simulink model "interlock_deadtime"  (R2020b)
settings: Solver=FixedStepDiscrete  StartTime=0.0  StopTime=0.01  RelTol=1e-3
libraries: eePwmGeneratorTwoLevel x1, powerlib_meascontrol x1, simulink x1, hdlsllib x1
settings Model: DataTypeOverride=Off  Creator=ts  LastModifiedBy=ts
settings DataIOCC: LimitDataPoints=on  SaveOutput=off  SaveTime=off
settings OptimizationCC: BlockReduction=off  ConditionallyExecuteInputs=off  DefaultParameterBehavior=Inlined  LifeSpan=inf
settings DebuggingCC: AlgebraicLoopMsg=error  SingleTaskRateTransMsg=error  AllowSymbolicDim=off  StrictBusMsg=ErrorOnBusTreatedAsVector  SFUnexpectedBacktrackingDiag=warning  SFNoUnconditionalDefaultTransitionDiag=warning  SFExecutionAtInitializationDiag=none  ArithmeticOperatorsInVariantConditions=warning
settings HardwareCC: ProdBitPerPointer=32  ProdBitPerSizeT=32  ProdBitPerPtrDiffT=32  ProdLargestAtomicFloat=None  ProdIntDivRoundTo=Undefined  ProdEndianess=Unspecified  ProdWordSize=32  ProdHWDeviceType=ASIC/FPGA->ASIC/FPGA  ProdEqTarget=off
settings SFSimCC: SimUseLocalCustomCode=off  CustomCodeUndefinedFunction=UseInterfaceOnly
settings RTWCC: RTWUseLocalCustomCode=off
settings CodeAppCC: StateflowObjectComments=on
settings GRTTargetCC: TargetLangStandard=C89/C90 (ANSI)
settings ConfigComp: CovScope=ReferencedModels  CovMetricSettings=dw  CovSaveCumulativeToWorkspaceVar=on  CovSaveSingleToWorkspaceVar=on  CovExternalEMLEnable=off  CovSFcnEnable=off

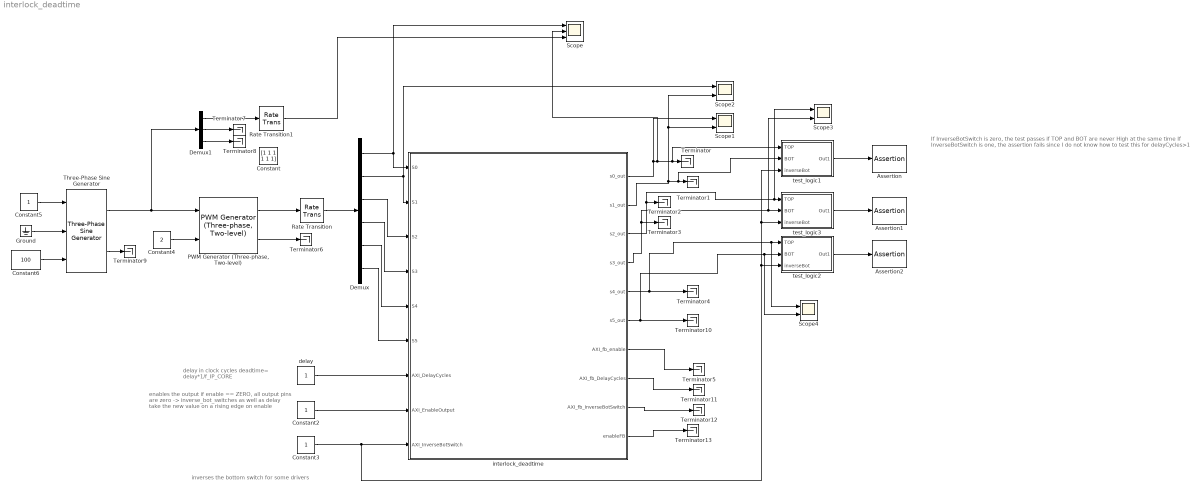
== system interlock_deadtime ==
  note: If InverseBotSwitch is zero, the test passes if TOP and BOT are never High at the same time
      | If InverseBotSwitch is one, the assertion fails since I do not know how to test this for delayCycles>1
  note: enables the output
      | if enable == ZERO, all output pins are zero
      |
      | -> inverse_bot_switches as well as delay take the
      | new value on a rising edge on enable
  note: inverses the bottom switch for some drivers
  note: delay in clock cycles
      | deadtime= delay*1/f_IP_CORE
  Assertion : Assertion
  Assertion1 : Assertion
  Assertion2 : Assertion
  Constant : Constant  Value=[1 1 1 1 1 1]  OutDataTypeStr=boolean
  Constant2 : Constant  OutDataTypeStr=boolean  SampleTime=1/100e6
  Constant3 : Constant  OutDataTypeStr=boolean  SampleTime=1/100e6
  Constant4 : Constant  Value=2  SampleTime=-1
  Constant5 : Constant  SampleTime=-1
  Constant6 : Constant  Value=100  SampleTime=-1
  Demux : Demux  Outputs=6
  Demux1 : Demux  Outputs=3
  Ground : Ground
  "PWM Generator (Three-phase, Two-level)" : eePwmGeneratorTwoLevel/PWM Generator (Three-phase, Two-level)  PWMMode=Continuous PWM (CPWM)  CPWMMode=SPWM: sinusoidal PWM  DPWMMode=60 DPWM: 60 degree discontinuous PWM  fsw=10e3  Ts=1/(100*100e3)
      settings: SourceProductBaseCode=PS
  Rate Transition : RateTransition  OutPortSampleTime=1/100e6
  Rate Transition1 : RateTransition  OutPortSampleTime=1/100e6
  Scope : Scope  NumInputPorts=3
  Scope{1..4} (4 alike) : Scope  NumInputPorts=2
  Terminator{,1..13} (14 alike) : Terminator
  Three-Phase Sine Generator : powerlib_meascontrol/Pulse & Signal Generators/Three-Phase Sine Generator  Ts=1/100e3
      settings: SourceProductBaseCode=PS
  delay : Constant  OutDataTypeStr=fixdt(0,10,0)  SampleTime=1/100e6
  interlock_deadtime : Subsystem  TreatAsAtomicUnit=on
  test_logic1 : Subsystem
  test_logic2 : Subsystem
  test_logic3 : Subsystem
  wires:
  Constant2/1 -> interlock_deadtime/8(AXI_EnableOutput)
  interlock_deadtime/1(s0_out) -> Scope/2, test_logic1/1(TOP), Terminator/1, Scope1/1
  interlock_deadtime/2(s1_out) -> Scope1/2, Scope2/2, test_logic1/2(BOT), Terminator1/1
  interlock_deadtime/3(s2_out) -> Scope3/1, test_logic3/1(TOP), Terminator2/1
  interlock_deadtime/4(s3_out) -> Scope3/2, test_logic3/2(BOT), Terminator3/1
  interlock_deadtime/5(s4_out) -> Scope4/1, test_logic2/1(TOP), Terminator4/1
  Constant4/1 -> "PWM Generator (Three-phase, Two-level)"/2
  Three-Phase Sine Generator/1 -> Demux1/1, "PWM Generator (Three-phase, Two-level)"/1
  Constant5/1 -> Three-Phase Sine Generator/1
  Constant6/1 -> Three-Phase Sine Generator/3
  Demux/1 -> Scope/1, interlock_deadtime/1(S0)
  Demux/2 -> Scope2/1, interlock_deadtime/2(S1)
  Demux/3 -> interlock_deadtime/3(S2)
  Demux/4 -> interlock_deadtime/4(S3)
  Demux/5 -> interlock_deadtime/5(S4)
  Demux/6 -> interlock_deadtime/6(S5)
  Demux1/1 -> Rate Transition1/1
  Rate Transition1/1 -> Scope/3
  Constant3/1 -> interlock_deadtime/9(AXI_InverseBotSwitch), test_logic2/3(inverseBot), test_logic3/3(inverseBot), test_logic1/3(inverseBot)
  "PWM Generator (Three-phase, Two-level)"/2 -> Terminator6/1
  Demux1/2 -> Terminator7/1
  Demux1/3 -> Terminator8/1
  Three-Phase Sine Generator/2 -> Terminator9/1
  Ground/1 -> Three-Phase Sine Generator/2
  interlock_deadtime/6(s5_out) -> Scope4/2, test_logic2/2(BOT), Terminator10/1
  interlock_deadtime/7(AXI_fb_enable) -> Terminator5/1
  interlock_deadtime/8(AXI_fb_DelayCycles) -> Terminator11/1
  interlock_deadtime/9(AXI_fb_InverseBotSwitch) -> Terminator12/1
  interlock_deadtime/10(enableFB) -> Terminator13/1
  test_logic3/1(Out1) -> Assertion1/1
  test_logic2/1(Out1) -> Assertion2/1
  test_logic1/1(Out1) -> Assertion/1
  Rate Transition/1 -> Demux/1
  "PWM Generator (Three-phase, Two-level)"/1 -> Rate Transition/1
  delay/1 -> interlock_deadtime/7(AXI_DelayCycles)

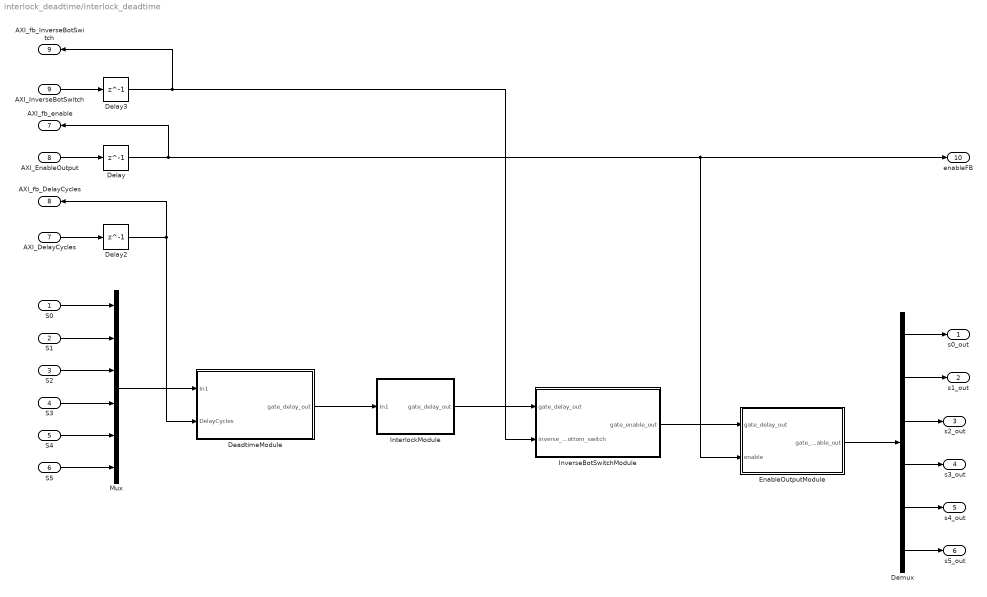
== system interlock_deadtime/interlock_deadtime ==
  S0 : Inport
  S1 : Inport  Port=2
  S2 : Inport  Port=3
  S3 : Inport  Port=4
  S4 : Inport  Port=5
  S5 : Inport  Port=6
  AXI_DelayCycles : Inport  Port=7
  AXI_EnableOutput : Inport  Port=8
  AXI_InverseBotSwitch : Inport  Port=9
  DeadtimeModule : Subsystem  TreatAsAtomicUnit=on
  Delay : Delay  DelayLength=1
  Delay2 : Delay  DelayLength=1
  Delay3 : Delay  DelayLength=1
  Demux : Demux  Outputs=6
  EnableOutputModule : Subsystem  TreatAsAtomicUnit=on
  InterlockModule : Subsystem  TreatAsAtomicUnit=on
  InverseBotSwitchModule : Subsystem  TreatAsAtomicUnit=on
  Mux : Mux  Inputs=6
  s0_out : Outport  VectorParamsAs1DForOutWhenUnconnected=off
  s1_out : Outport  Port=2  VectorParamsAs1DForOutWhenUnconnected=off
  s2_out : Outport  Port=3  VectorParamsAs1DForOutWhenUnconnected=off
  s3_out : Outport  Port=4  VectorParamsAs1DForOutWhenUnconnected=off
  s4_out : Outport  Port=5  VectorParamsAs1DForOutWhenUnconnected=off
  s5_out : Outport  Port=6  VectorParamsAs1DForOutWhenUnconnected=off
  AXI_fb_enable : Outport  Port=7  VectorParamsAs1DForOutWhenUnconnected=off
  AXI_fb_DelayCycles : Outport  Port=8  VectorParamsAs1DForOutWhenUnconnected=off
  AXI_fb_InverseBotSwitch : Outport  Port=9  VectorParamsAs1DForOutWhenUnconnected=off
  enableFB : Outport  Port=10  VectorParamsAs1DForOutWhenUnconnected=off
  wires:
  AXI_InverseBotSwitch/1 -> Delay3/1
  Delay3/1 -> InverseBotSwitchModule/2(inverse_bottom_switch), AXI_fb_InverseBotSwitch/1
  AXI_EnableOutput/1 -> Delay/1
  Delay2/1 -> AXI_fb_DelayCycles/1, DeadtimeModule/2(DelayCycles)
  Mux/1 -> DeadtimeModule/1(In1)
  DeadtimeModule/1(gate_delay_out) -> InterlockModule/1(In1)
  S0/1 -> Mux/1
  S1/1 -> Mux/2
  S2/1 -> Mux/3
  S3/1 -> Mux/4
  S4/1 -> Mux/5
  S5/1 -> Mux/6
  Demux/2 -> s1_out/1
  Demux/1 -> s0_out/1
  Demux/3 -> s2_out/1
  Demux/4 -> s3_out/1
  Demux/5 -> s4_out/1
  Demux/6 -> s5_out/1
  EnableOutputModule/1(gate_enable_out) -> Demux/1
  Delay/1 -> AXI_fb_enable/1, enableFB/1, EnableOutputModule/2(enable)
  InterlockModule/1(gate_delay_out) -> InverseBotSwitchModule/1(gate_delay_out)
  InverseBotSwitchModule/1(gate_enable_out) -> EnableOutputModule/1(gate_delay_out)
  AXI_DelayCycles/1 -> Delay2/1

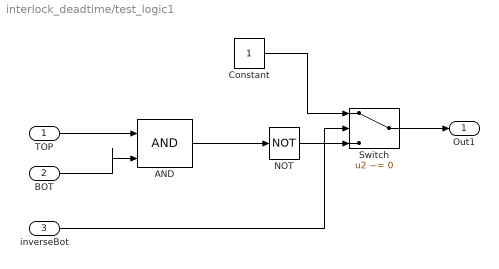
== system interlock_deadtime/test_logic1 ==
  TOP : Inport
  BOT : Inport  Port=2
  inverseBot : Inport  Port=3
  AND : Logic  IconShape=distinctive  AllPortsSameDT=off  OutDataTypeStr=boolean
  Constant : Constant
  NOT : Logic  Operator=NOT  IconShape=distinctive  AllPortsSameDT=off  OutDataTypeStr=boolean
  Switch : Switch  Criteria=u2 ~= 0
  Out1 : Outport
  wires:
  Constant/1 -> Switch/1
  Switch/1 -> Out1/1
  AND/1 -> NOT/1
  inverseBot/1 -> Switch/2
  NOT/1 -> Switch/3
  TOP/1 -> AND/1
  BOT/1 -> AND/2

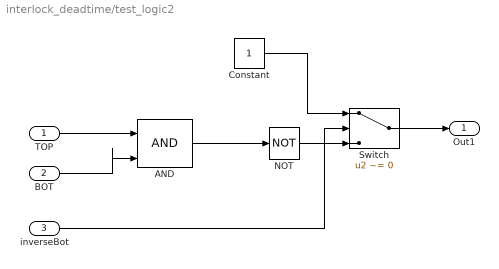
== system interlock_deadtime/test_logic2 ==
  TOP : Inport
  BOT : Inport  Port=2
  inverseBot : Inport  Port=3
  AND : Logic  IconShape=distinctive  AllPortsSameDT=off  OutDataTypeStr=boolean
  Constant : Constant
  NOT : Logic  Operator=NOT  IconShape=distinctive  AllPortsSameDT=off  OutDataTypeStr=boolean
  Switch : Switch  Criteria=u2 ~= 0
  Out1 : Outport
  wires:
  BOT/1 -> AND/2
  TOP/1 -> AND/1
  NOT/1 -> Switch/3
  inverseBot/1 -> Switch/2
  AND/1 -> NOT/1
  Switch/1 -> Out1/1
  Constant/1 -> Switch/1

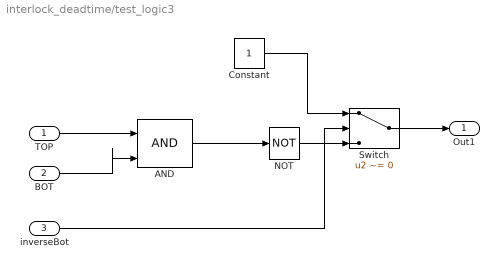
== system interlock_deadtime/test_logic3 ==
  TOP : Inport
  BOT : Inport  Port=2
  inverseBot : Inport  Port=3
  AND : Logic  IconShape=distinctive  AllPortsSameDT=off  OutDataTypeStr=boolean
  Constant : Constant
  NOT : Logic  Operator=NOT  IconShape=distinctive  AllPortsSameDT=off  OutDataTypeStr=boolean
  Switch : Switch  Criteria=u2 ~= 0
  Out1 : Outport
  wires:
  Constant/1 -> Switch/1
  Switch/1 -> Out1/1
  AND/1 -> NOT/1
  inverseBot/1 -> Switch/2
  NOT/1 -> Switch/3
  TOP/1 -> AND/1
  BOT/1 -> AND/2

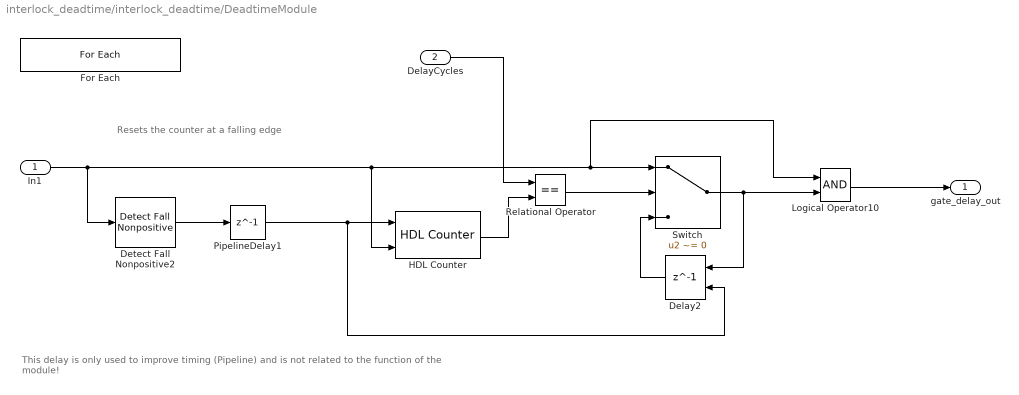
== system interlock_deadtime/interlock_deadtime/DeadtimeModule ==
  note: Resets the counter at a falling edge
  note: This delay is only used to improve timing (Pipeline) and is not related to the function of the module!
  In1 : Inport  Partition=on  PartitionDimension=1  PartitionWidth=1  PartitionOffset=0
  DelayCycles : Inport  Port=2
  Delay2 : Delay  DelayLength=1  ExternalReset=Level
      settings: InputPortMap=u0,r5
  Detect Fall Nonpositive2 : simulink/Logic and Bit Operations/Detect Fall Nonpositive  vinit=0  OutDataTypeStr=boolean
      settings: SourceProductBaseCode=SL
  For Each : ForEach  DisableCoverage=on
  HDL Counter : hdlsllib/Sources/HDL Counter  CountType=Free running  CountInit=0  CountStep=1  CountMax=25  CountFromType=Initial value  CountFrom=0  CountResetPort=on  CountLoadPort=off  CountEnbPort=on  CountDirPort=off  CountDataType=Unsigned  CountWordLen=10  CountFracLen=0  CountSampTime=-1
  Logical Operator10 : Logic  AllPortsSameDT=off  OutDataTypeStr=boolean
  PipelineDelay1 : Delay  DelayLength=1
  Relational Operator : RelationalOperator  Operator===  OutDataTypeStr=boolean  RndMeth=Simplest
  Switch : Switch  Criteria=u2 ~= 0  Threshold=1
  gate_delay_out : Outport  ConcatenationDimension=1
  wires:
  In1/1 -> Logical Operator10/1, Switch/1, HDL Counter/2, Detect Fall Nonpositive2/1
  DelayCycles/1 -> Relational Operator/1
  Delay2/1 -> Switch/3
  HDL Counter/1 -> Relational Operator/2
  Detect Fall Nonpositive2/1 -> PipelineDelay1/1
  Relational Operator/1 -> Switch/2
  PipelineDelay1/1 -> HDL Counter/1, Delay2/2
  Switch/1 -> Delay2/1, Logical Operator10/2
  Logical Operator10/1 -> gate_delay_out/1

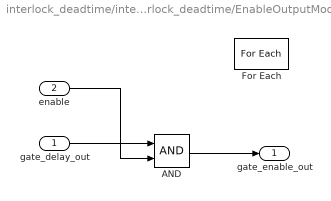
== system interlock_deadtime/interlock_deadtime/EnableOutputModule ==
  gate_delay_out : Inport  Partition=on  PartitionDimension=1  PartitionWidth=1  PartitionOffset=0
  enable : Inport  Port=2
  AND : Logic  AllPortsSameDT=off  OutDataTypeStr=boolean
  For Each : ForEach  DisableCoverage=on
  gate_enable_out : Outport  ConcatenationDimension=1
  wires:
  enable/1 -> AND/2
  gate_delay_out/1 -> AND/1
  AND/1 -> gate_enable_out/1

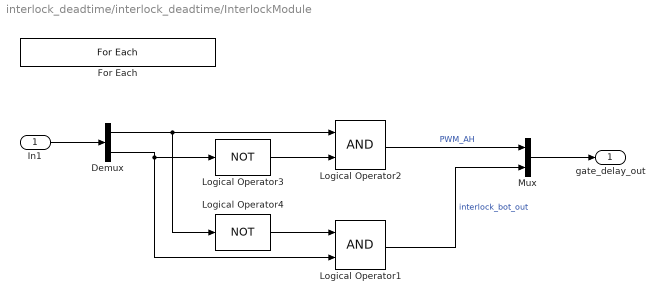
== system interlock_deadtime/interlock_deadtime/InterlockModule ==
  In1 : Inport  Partition=on  PartitionDimension=1  PartitionWidth=2  PartitionOffset=0
  Demux : Demux  Outputs=2
  For Each : ForEach  DisableCoverage=on
  Logical Operator1 : Logic  AllPortsSameDT=off  OutDataTypeStr=boolean
  Logical Operator2 : Logic  AllPortsSameDT=off  OutDataTypeStr=boolean
  Logical Operator3 : Logic  Operator=NOT  AllPortsSameDT=off  OutDataTypeStr=boolean
  Logical Operator4 : Logic  Operator=NOT  AllPortsSameDT=off  OutDataTypeStr=boolean
  Mux : Mux  Inputs=2
  gate_delay_out : Outport  ConcatenationDimension=1
  wires:
  Demux/1 -> Logical Operator4/1, Logical Operator2/1
  Logical Operator1/1 -> Mux/2  "interlock_bot_out"
  Demux/2 -> Logical Operator1/2, Logical Operator3/1
  Logical Operator3/1 -> Logical Operator2/2
  Logical Operator2/1 -> Mux/1  "PWM_AH"
  Logical Operator4/1 -> Logical Operator1/1
  Mux/1 -> gate_delay_out/1
  In1/1 -> Demux/1

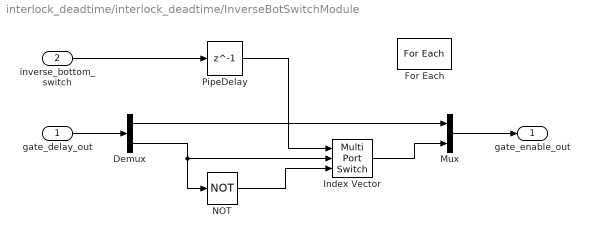
== system interlock_deadtime/interlock_deadtime/InverseBotSwitchModule ==
  gate_delay_out : Inport  Partition=on  PartitionDimension=1  PartitionWidth=2  PartitionOffset=0
  inverse_bottom_switch : Inport  Port=2
  Demux : Demux  Outputs=2
  For Each : ForEach  DisableCoverage=on
  Index Vector : MultiPortSwitch  DataPortOrder=Zero-based contiguous  Inputs=2  zeroidx=on
  Mux : Mux  Inputs=2
  NOT : Logic  Operator=NOT  AllPortsSameDT=off  OutDataTypeStr=boolean
  PipeDelay : Delay  DelayLength=1
  gate_enable_out : Outport  ConcatenationDimension=1
  wires:
  PipeDelay/1 -> Index Vector/1
  Demux/2 -> Index Vector/2, NOT/1
  Index Vector/1 -> Mux/2
  inverse_bottom_switch/1 -> PipeDelay/1
  Demux/1 -> Mux/1
  NOT/1 -> Index Vector/3
  Mux/1 -> gate_enable_out/1
  gate_delay_out/1 -> Demux/1
